simulink model "modeloPerturbacion"  (R2024b)
settings: Solver=VariableStepAuto  StartTime=0.0  StopTime=10.0  RelTol=1e-3
settings Model: Creator=estel  LastModifiedBy=estel

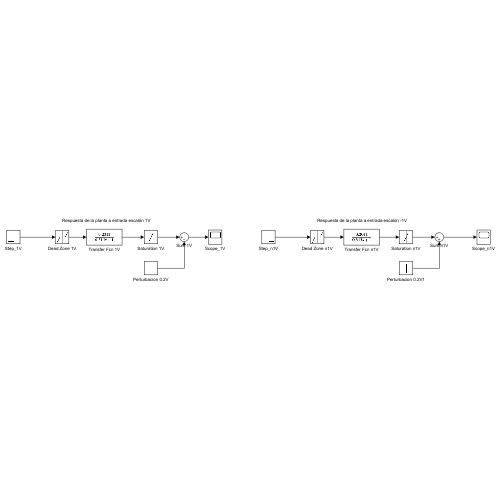
[thumbnail: Simulink's stored preview of the top-level diagram]
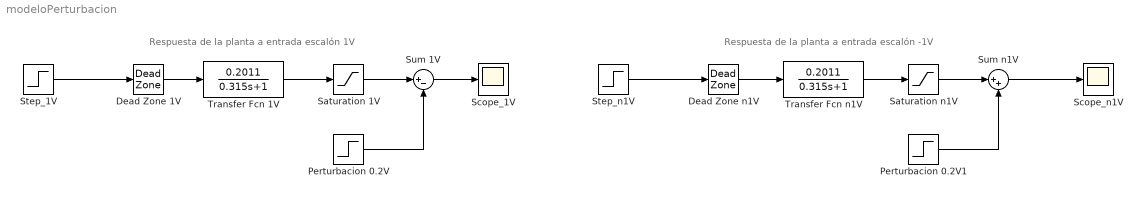
== system modeloPerturbacion ==
  note: Respuesta de la planta a entrada escalón 1V
  note: Respuesta de la planta a entrada escalón -1V
  Dead Zone 1V : DeadZone  LowerValue=-0.19  UpperValue=0.19
  Dead Zone n1V : DeadZone  LowerValue=-0.19  UpperValue=0.19
  Perturbacion 0.2V : Step  Time=5  After=0.2  SampleTime=0
  Perturbacion 0.2V1 : Step  Time=5  After=0.2  SampleTime=0
  Saturation 1V : Saturate  UpperLimit=10  LowerLimit=-10
  Saturation n1V : Saturate  UpperLimit=10  LowerLimit=-10
  Scope_1V : Scope
  Scope_n1V : Scope
  Step_1V : Step  SampleTime=0
  Step_n1V : Step  After=-1  SampleTime=0
  Sum 1V : Sum  Inputs=|+-
  Sum n1V : Sum  Inputs=|++
  Transfer Fcn 1V : TransferFcn  Numerator=0.2011  Denominator=[0.315 1]
  Transfer Fcn n1V : TransferFcn  Numerator=0.2011  Denominator=[0.315 1]
  wires:
  Transfer Fcn 1V/1 -> Saturation 1V/1
  Step_1V/1 -> Dead Zone 1V/1
  Dead Zone 1V/1 -> Transfer Fcn 1V/1
  Dead Zone n1V/1 -> Transfer Fcn n1V/1
  Step_n1V/1 -> Dead Zone n1V/1
  Transfer Fcn n1V/1 -> Saturation n1V/1
  Saturation n1V/1 -> Sum n1V/1
  Saturation 1V/1 -> Sum 1V/1
  Perturbacion 0.2V/1 -> Sum 1V/2
  Sum 1V/1 -> Scope_1V/1
  Perturbacion 0.2V1/1 -> Sum n1V/2
  Sum n1V/1 -> Scope_n1V/1
